simulink model "rocket_dynamics_hybrid"  (R2024b)
settings: Solver=VariableStepAuto  StartTime=0.0  StopTime=30000  RelTol=1e-3
PreLoadFcn:
  | run("rocket_init.m");
values from neighbouring files (symbols this model uses):
  A = 1.0    (= 1)    [rocket_init.m]
  ballistic = false    [rocket_init.m]
  Cd = 0.5    [rocket_init.m]
  Cl = 0.4    [rocket_init.m]
  m0 = mrc0 + mf0    (= 1100)    [rocket_init.m]
  m_dot = 5    [rocket_init.m]
  mrc0 = 1000    [rocket_init.m]
  r0 = h0 + Re    (= 6371000)    [rocket_init.m]
  Re = 6.371e6    (= 6371000)    [rocket_init.m]
  Vr0 = 0    [rocket_init.m]
  Vv0 = 0    [rocket_init.m]
libraries: simulink_extras x1
settings Model: Creator=gabor  LastModifiedBy=gabor
settings DebuggingCC: UnderSpecifiedDimensionMsg=warning

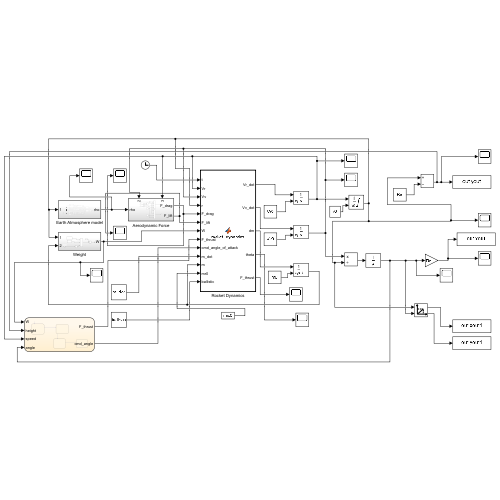
[thumbnail: Simulink's stored preview of the top-level diagram]
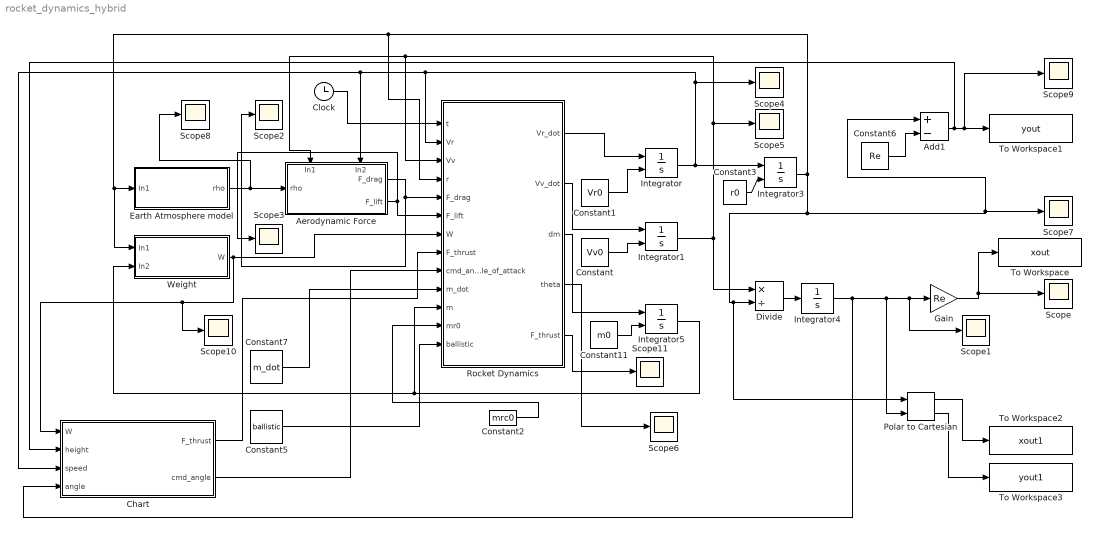
== system rocket_dynamics_hybrid ==
  Add1 : Sum  Inputs=+-
  Aerodynamic Force : Subsystem
      settings: PortSchema="{\"entries\":[{\"content\":{\"sides\":[{\"content\":{\"connectorIds\":[\"In1\"]},\"type\":\"ConnectorPlacement.EquallySpacedRectSide\",\"uuid\":\"72e9719d-e03c-4d33-84d7-0d4ee9582499\"},{\"content\":{\"connectorIds\":[\"Out1\",\"Out2\"],\"side\":\"RIGHT\"},\"type\":\"ConnectorPlacement.EquallySpacedRectSide\",\"uuid\":\"f4b6d6a9-ab34-4dcc-96f7-09b22e6a40b3\"},{\"content\":{\"connectorIds\":[\"In2\",\"In3\"],\"side\":\"TOP\"},\"type\":\"ConnectorPlacement.EquallySpacedRectSide\",\"uuid\":\"1597c7e2-1455-4607-8e57-0d7b41b5dcd7\"}]},\"type\":\"ConnectorPlacement.EquallySpacedConnector\",\"uuid\":\"e5b19b30-5e08-4bac-afeb-f99624a6d39d\"}],\"packageUris\":[\"http://schema.mathworks.com/mf0/Connector/R2020b\"],\"version\":\"1.0\"}"
  Chart : Stateflow chart  TreatAsAtomicUnit=on
      settings: PortSchema="{\"entries\":[{\"content\":{\"sides\":[{\"content\":{\"connectorIds\":[\"In2\",\"In1\",\"In3\",\"In4\"]},\"type\":\"ConnectorPlacement.EquallySpacedRectSide\",\"uuid\":\"83da7449-999a-4ed0-986b-73ec89efc96f\"},{\"content\":{\"connectorIds\":[\"Out1\",\"Out2\"],\"side\":\"RIGHT\"},\"type\":\"ConnectorPlacement.EquallySpacedRectSide\",\"uuid\":\"9dcd0efc-068d-4e48-b250-d887bf0aea2b\"},{\"content\":{\"side\":\"TOP\"},\"type\":\"ConnectorPlacement.EquallySpacedRectSide\",\"uuid\":\"87b3b07d-3da2-4b71-91c9-fb2ce18483c4\"}]},\"type\":\"ConnectorPlacement.EquallySpacedConnector\",\"uuid\":\"093ee1b0-d816-4ab5-9c4c-f62d21b68a3f\"}],\"packageUris\":[\"http://schema.mathworks.com/mf0/Connector/R2020b\"],\"version\":\"1.0\"}"
  Clock : Clock
  Constant : Constant  Value=Vv0
  Constant1 : Constant  Value=Vr0
  Constant11 : Constant  Value=m0
  Constant2 : Constant  Value=mrc0
  Constant3 : Constant  Value=r0
  Constant5 : Constant  Value=ballistic
  Constant6 : Constant  Value=Re
  Constant7 : Constant  Value=m_dot
  Divide : Product  Inputs=*/
  Earth Atmosphere model : Subsystem
  Gain : Gain  Gain=Re
  Integrator : Integrator  InitialConditionSource=external
  Integrator1 : Integrator  InitialConditionSource=external  LowerSaturationLimit=0
  Integrator3 : Integrator  InitialConditionSource=external  LimitOutput=on  LowerSaturationLimit=Re
  Integrator4 : Integrator  LowerSaturationLimit=0
  Integrator5 : Integrator  InitialConditionSource=external  LimitOutput=on  LowerSaturationLimit=mrc0
  Polar to Cartesian : simulink_extras/Transformations/Polar to Cartesian
  Rocket Dynamics : MATLAB Function  TreatAsAtomicUnit=on
  Scope{,1..11} (12 alike) : Scope
  To Workspace : ToWorkspace  VariableName=xout  SaveFormat=Timeseries  SampleTime=-1
  To Workspace1 : ToWorkspace  VariableName=yout  SaveFormat=Timeseries  SampleTime=-1
  To Workspace2 : ToWorkspace  VariableName=xout1  SaveFormat=Timeseries  SampleTime=-1
  To Workspace3 : ToWorkspace  VariableName=yout1  SaveFormat=Timeseries  SampleTime=-1
  Weight : Subsystem
  wires:
  Rocket Dynamics/1(Vr_dot) -> Integrator/1
  Rocket Dynamics/2(Vv_dot) -> Integrator1/1
  Integrator/1 -> Integrator3/1, Scope4/1, Rocket Dynamics/2(Vr), Aerodynamic Force/3(In2), Chart/3(speed)
  Integrator1/1 -> Divide/1, Scope5/1, Aerodynamic Force/2(In1), Rocket Dynamics/3(Vv)
  Rocket Dynamics/3(dm) -> Integrator5/1
  Constant/1 -> Integrator1/2
  Constant1/1 -> Integrator/2
  Constant11/1 -> Integrator5/2
  Constant3/1 -> Integrator3/2
  Integrator5/1 -> Weight/2(In2), Rocket Dynamics/11(m)
  Aerodynamic Force/1(F_drag) -> Scope2/1, Rocket Dynamics/5(F_drag)
  Aerodynamic Force/2(F_lift) -> Scope3/1, Rocket Dynamics/6(F_lift)
  Weight/1(W) -> Chart/2(W), Scope10/1, Rocket Dynamics/7(W)
  Constant7/1 -> Rocket Dynamics/10(m_dot)
  Constant2/1 -> Rocket Dynamics/12(mr0)
  Rocket Dynamics/4(theta) -> Scope6/1
  Clock/1 -> Rocket Dynamics/1(t)
  Integrator3/1 -> Add1/1, Scope7/1, Polar to Cartesian/1, Divide/2, Weight/1(In1), Earth Atmosphere model/1(In1), Rocket Dynamics/4(r)
  Constant6/1 -> Add1/2
  Add1/1 -> Chart/1(height), Scope9/1, To Workspace1/1
  Gain/1 -> To Workspace/1, Scope/1
  Integrator4/1 -> Polar to Cartesian/2, Scope1/1, Gain/1, Chart/4(angle)
  Constant5/1 -> Rocket Dynamics/13(ballistic)
  Divide/1 -> Integrator4/1
  Earth Atmosphere model/1(rho) -> Scope8/1, Aerodynamic Force/1(rho)
  Polar to Cartesian/1 -> To Workspace2/1
  Polar to Cartesian/2 -> To Workspace3/1
  Rocket Dynamics/5(F_thrust) -> Scope11/1
  Chart/1(F_thrust) -> Rocket Dynamics/8("F_thrust ")
  Chart/2(cmd_angle) -> Rocket Dynamics/9(cmd_angle_of_attack)

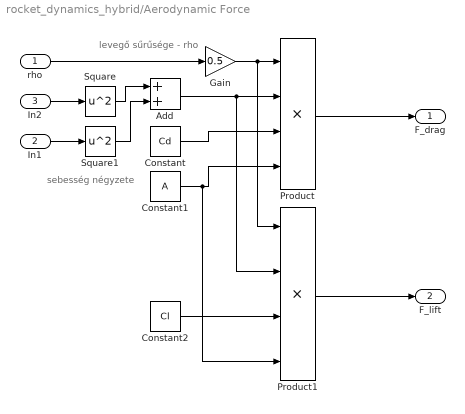
== system rocket_dynamics_hybrid/Aerodynamic Force ==
  note: levegő sűrűsége - rho
  note: sebesség négyzete
  rho : Inport
  In1 : Inport  Port=2
  In2 : Inport  Port=3
  Add : Sum
  Constant : Constant  Value=Cd
  Constant1 : Constant  Value=A
  Constant2 : Constant  Value=Cl
  Gain : Gain  Gain=0.5
  Product : Product  Inputs=4
  Product1 : Product  Inputs=4
  Square : Math  Operator=square
  Square1 : Math  Operator=square
  F_drag : Outport
  F_lift : Outport  Port=2
  wires:
  rho/1 -> Gain/1
  Gain/1 -> Product1/1, Product/1
  Constant/1 -> Product/3
  Constant1/1 -> Product1/4, Product/4
  Product/1 -> F_drag/1
  In2/1 -> Square/1
  In1/1 -> Square1/1
  Square/1 -> Add/1
  Square1/1 -> Add/2
  Add/1 -> Product1/2, Product/2
  Constant2/1 -> Product1/3
  Product1/1 -> F_lift/1

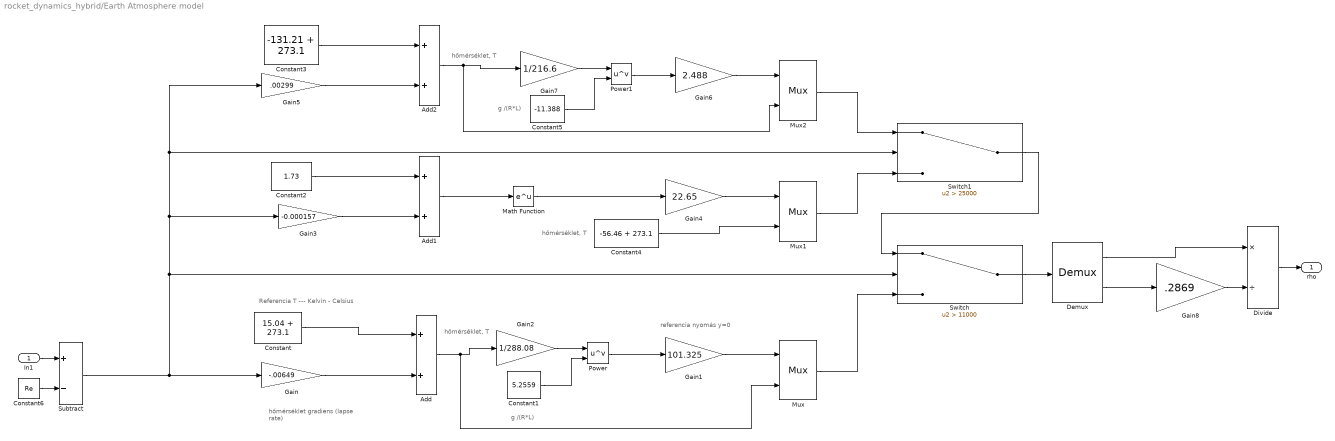
== system rocket_dynamics_hybrid/Earth Atmosphere model ==
  note: g /(R*L)
  note: referencia nyomás y=0
  note: Referencia T --- Kelvin - Celsius
  note: hőmérséklet, T
  note: hőmérséklet gradiens
      | (lapse rate)
  note: g /(R*L)
  note: hőmérséklet, T
  note: hőmérséklet, T
  In1 : Inport
  Add : Sum
  Add1 : Sum
  Add2 : Sum
  Constant : Constant  Value=15.04 + 273.1
  Constant1 : Constant  Value=5.2559
  Constant2 : Constant  Value=1.73
  Constant3 : Constant  Value=-131.21 + 273.1
  Constant4 : Constant  Value=-56.46 + 273.1
  Constant5 : Constant  Value=-11.388
  Constant6 : Constant  Value=Re
  Demux : Demux  Outputs=2
      settings: DisplayOption=none
  Divide : Product  Inputs=*/
  Gain : Gain  Gain=-.00649
  Gain1 : Gain  Gain=101.325
  Gain2 : Gain  Gain=1/288.08
  Gain3 : Gain  Gain=-0.000157
  Gain4 : Gain  Gain=22.65
  Gain5 : Gain  Gain=.00299
  Gain6 : Gain  Gain=2.488
  Gain7 : Gain  Gain=1/216.6
  Gain8 : Gain  Gain=.2869
  Math Function : Math
  Mux : Mux  Inputs=2
  Mux1 : Mux  Inputs=2
  Mux2 : Mux  Inputs=2
  Power : Math  Operator=pow
  Power1 : Math  Operator=pow
  Subtract : Sum  Inputs=+-
  Switch : Switch  Criteria=u2 > Threshold  Threshold=11000  SaturateOnIntegerOverflow=off  InputSameDT=off
  Switch1 : Switch  Criteria=u2 > Threshold  Threshold=25000  SaturateOnIntegerOverflow=off  InputSameDT=off
  rho : Outport
  wires:
  Subtract/1 -> Switch/2, Gain5/1, Switch1/2, Gain3/1, Gain/1
  Gain/1 -> Add/2
  Add/1 -> Mux/2, Gain2/1
  Gain2/1 -> Power/1
  Constant1/1 -> Power/2
  Power/1 -> Gain1/1
  Gain3/1 -> Add1/2
  Add1/1 -> Math Function/1
  Math Function/1 -> Gain4/1
  Constant/1 -> Add/1
  Constant2/1 -> Add1/1
  Constant3/1 -> Add2/1
  Gain5/1 -> Add2/2
  Gain7/1 -> Power1/1
  Constant5/1 -> Power1/2
  Power1/1 -> Gain6/1
  Add2/1 -> Mux2/2, Gain7/1
  Gain1/1 -> Mux/1
  Gain4/1 -> Mux1/1
  Constant4/1 -> Mux1/2
  Gain6/1 -> Mux2/1
  Mux/1 -> Switch/3
  Mux1/1 -> Switch1/3
  Mux2/1 -> Switch1/1
  Switch1/1 -> Switch/1
  Switch/1 -> Demux/1
  Demux/2 -> Gain8/1
  Gain8/1 -> Divide/2
  Demux/1 -> Divide/1
  Divide/1 -> rho/1
  Constant6/1 -> Subtract/2
  In1/1 -> Subtract/1

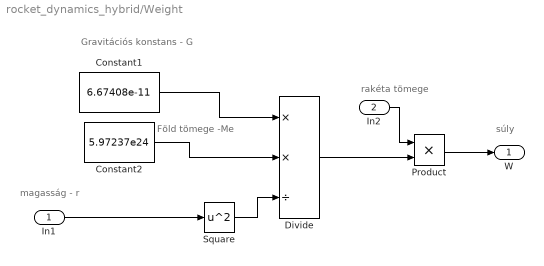
== system rocket_dynamics_hybrid/Weight ==
  note: rakéta tömege
  note: súly
  note: Gravitációs konstans - G
  note: magasság - r
  note: Föld tömege -Me
  In1 : Inport
  In2 : Inport  Port=2
  Constant1 : Constant  Value=6.67408e-11
  Constant2 : Constant  Value=5.97237e24
  Divide : Product  Inputs=**/
  Product : Product
  Square : Math  Operator=square
  W : Outport
  wires:
  Square/1 -> Divide/3
  Constant1/1 -> Divide/1
  Constant2/1 -> Divide/2
  In2/1 -> Product/1
  Divide/1 -> Product/2
  Product/1 -> W/1
  In1/1 -> Square/1

== matlab function rocket_dynamics_hybrid/Rocket Dynamics ==
  data: t input; Vr input; Vv input; r input; F_drag input; F_lift input; W input; F_thrust input; cmd_angle_of_attack input; Vr_dot output; Vv_dot output; m_dot input; m input; dm output; mr0 input; theta output; ballistic input; F_thrust output
function [Vr_dot,Vv_dot,dm,theta,F_thrust] = rocket_dynamics(t,Vr,Vv,r,F_drag,F_lift,W,F_thrust,cmd_angle_of_attack,m_dot,m,mr0,ballistic)
% Rakéta dinamikai modell

vel_angle = atan2(Vr,Vv);

theta = cmd_angle_of_attack;

if(ballistic)
    Vr_dot = (Vv^2)/r + (-F_drag*sin(vel_angle)+F_thrust*sin(theta) - W)/m;
    Vv_dot = -(Vr*Vv)/r - (F_drag*cos(vel_angle) - F_thrust*cos(theta))/m;
else
    Vr_dot = (Vv^2)/r + (F_lift*cos(vel_angle)-F_drag*sin(vel_angle)+F_thrust*sin(theta) - W)/m;
    Vv_dot = -(Vr*Vv)/r - (F_lift*sin(vel_angle) + F_drag*cos(vel_angle) - F_thrust*cos(theta))/m;
end

dm = -m_dot;


end

== stateflow chart rocket_dynamics_hybrid/Chart ==
  state Boost
    entry:
    cmd_angle = deg2rad(80);
    F_thrust = W;
    during:
    F_thrust = F_thrust + 200;
  state Speed_reached
    %Stop increasing Thrust
    %Maintain Speed
  state Turn
    entry:
    cmd_angle = 0;
    F_thrust = F_thrust/4.2;
  state Stop_Thrust
    %Stop Thrust Force
    entry:
    F_thrust = 0;
  (default) -> Boost
  Boost -> Speed_reached : [speed > 1000]
  Speed_reached -> Turn : [height > 430000]
  Turn -> Stop_Thrust : [angle >= 0.51]
  data: height input; W input; F_thrust output; cmd_angle output; speed input; angle input
